simulink model "Opticflowtest_mod"  (Simulink 7.6)
settings: Solver=ode45  StartTime=0.0  StopTime=inf  RelTol=1e-3
undefined symbols (not defined in the file): Horn, none, Schunck, videoinput
libraries: dspstat3 x2, vipanalysis x2, imaqlib x1, simulink x1
settings Model: Creator=pacifist  LastModifiedBy=Administrator
settings SimEventsCC: propDiagAttribOutput=1  propDiagFcnCallOutput=1  propDiagStatOutput=0

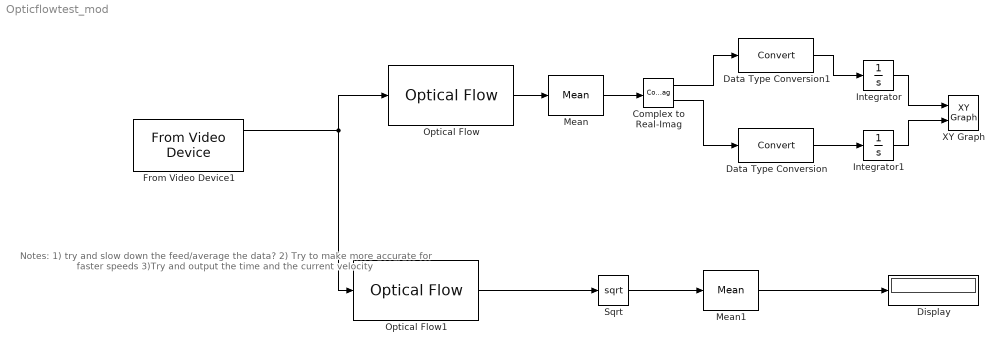
== system Opticflowtest_mod ==
  note: Notes:
      | 1) try and slow down the feed/average the data?
      | 2) Try to make more accurate for faster speeds
      | 3)Try and output the time and the current velocity
  Complex to Real-Imag : ComplexToRealImag
  Data Type Conversion : DataTypeConversion
  Data Type Conversion1 : DataTypeConversion
  Display : Display
  From Video Device1 : imaqlib/From Video Device  DialogController=imaqcreatedialog  DialogControllerArgs=DataTag1  DeviceMenu=winvideo 1 (VC0334 USB2.0 Digital Camera)  Device=linuxvideo 1 (UVC Camera (046d:0804))  ObjConstructor=videoinput('linuxvideo', 1)  VideoFormatMenu=RGB24_640x480  VideoFormat=YUYV_160x120  VideoSource=Camera 1  ROIPosition=[0 0 120 160]  EnableHWTrigger=off  TriggerConfiguration=none/none  SampleTime=1/30  OutputPortsMode=Separate color signals  DataType=single  CanDoHWTrigger=no  ReturnedColorSpace=YCbCr  BlockHandle=8.0013  ROIWidth=160  ROIHeight=120  ROIColumn=0  ROIRow=0  EngXMLPath=C:\Program Files\MATLAB\R2010b\toolbox\imaq\imaq\private  DevXMLPath=C:\Program Files\MATLAB\R2010b\toolbox\imaq\imaqadaptors\win32  EngLibPath=C:\Program Files\MATLAB\R2010b\toolbox\imaq\imaqblks\imaqmex\win32
  Integrator : Integrator
  Integrator1 : Integrator
  Mean : dspstat3/Mean  DialogController=dspDDGCreate  DialogControllerArgs=DataTag3  run=off  reset_popup=None  directionMode=Entire input  dimension=1  treatSBRowAsCol=on  roiEnable=off  roiType=Rectangles  roiPortion=Entire ROI  roiOutput=Individual statistics for each ROI  roiFlag=off  outputDataTypeStr=Inherit: Same as accumulator  outputLastDataTypeStr=Inherit: Same as accumulator  outputMin=[]  outputMax=[]  accumMode=Binary point scaling  accumWordLength=32  accumFracLength=0  accumDataTypeStr=fixdt([],32,0)  accumLastDataTypeStr=fixdt([],32,0)  roundingMode=Floor  overflowMode=off
  Mean1 : dspstat3/Mean  DialogController=dspDDGCreate  DialogControllerArgs=DataTag5  run=off  reset_popup=None  directionMode=Entire input  dimension=1  treatSBRowAsCol=on  roiEnable=off  roiType=Rectangles  roiPortion=Entire ROI  roiOutput=Individual statistics for each ROI  roiFlag=off  outputDataTypeStr=Inherit: Same as accumulator  outputLastDataTypeStr=Inherit: Same as accumulator  outputMin=[]  outputMax=[]  accumMode=Binary point scaling  accumWordLength=32  accumFracLength=0  accumDataTypeStr=fixdt([],32,0)  accumLastDataTypeStr=fixdt([],32,0)  roundingMode=Floor  overflowMode=off
  Optical Flow : vipanalysis/Optical Flow  DialogController=vipDDGCreate  DialogControllerArgs=DataTag6  SystemSampleTime=-1  method=Horn-Schunck  gradMethod=Difference filter [-1 1]  which2img=Current frame and N-th frame back  N=1  outVelForm=Horizontal and vertical components in complex form  lambda=5  stop_criteria=When maximum number of iterations is reached  maxAllowAbsDiff=eps  maxIter=10  numInports=3  sigmaS=1.5  sigmaW=1  eigTh=0.0039  discardNormalFlow=off  outputCurrentImage=off  prodOutputMode=Binary point scaling  prodOutputWordLength=32  prodOutputFracLength=20  outputMode=Binary point scaling  outputWordLength=32  outputFracLength=20  roundingMode=Nearest  overflowMode=on
      link override Optical Flow Estimation: which2img=Current frame and N-th frame back  outVelForm=Magnitude-squared
  Optical Flow1 : vipanalysis/Optical Flow  DialogController=vipDDGCreate  DialogControllerArgs=DataTag7  SystemSampleTime=-1  method=Horn-Schunck  gradMethod=Difference filter [-1 1]  which2img=Current frame and N-th frame back  N=1  outVelForm=Magnitude-squared  lambda=5  stop_criteria=When maximum number of iterations is reached  maxAllowAbsDiff=eps  maxIter=10  numInports=3  sigmaS=1.5  sigmaW=1  eigTh=0.0039  discardNormalFlow=off  outputCurrentImage=off  prodOutputMode=Binary point scaling  prodOutputWordLength=32  prodOutputFracLength=20  outputMode=Binary point scaling  outputWordLength=32  outputFracLength=20  roundingMode=Nearest  overflowMode=on
      link override Optical Flow Estimation: which2img=Current frame and N-th frame back  outVelForm=Magnitude-squared
  Sqrt : Sqrt  SaturateOnIntegerOverflow=on
  XY Graph : simulink/Sinks/XY Graph  SystemSampleTime=-1  xmin=-.01  xmax=.01  ymin=-.01  ymax=.01  st=-1
  wires:
  Optical Flow/1 -> Mean/1
  Mean/1 -> Complex to Real-Imag/1
  Complex to Real-Imag/1 -> Data Type Conversion1/1
  Complex to Real-Imag/2 -> Data Type Conversion/1
  Data Type Conversion/1 -> Integrator1/1
  Integrator1/1 -> XY Graph/2
  Data Type Conversion1/1 -> Integrator/1
  Integrator/1 -> XY Graph/1
  Optical Flow1/1 -> Sqrt/1
  From Video Device1/1 -> Optical Flow1/1, Optical Flow/1
  Sqrt/1 -> Mean1/1
  Mean1/1 -> Display/1
